simulink model "generalized_plant"  (R2023b)
settings: Solver=VariableStepAuto  StartTime=0.0  StopTime=10.0  RelTol=1e-3
values from neighbouring files (symbols this model uses):
  G_a = 0.095    [Problem_1.m]    (also in Problem_2.m = -0.09; Problem_3.m = 0.014; Problem_4.m = 0.006; Problem_5.m = 0.38)
  G_f = 1 / (K_d*G_s)    (= 1)    [Problem_1.m]    (also in Problem_2.m; Problem_3.m; Problem_4.m; Problem_5.m = 0.125)
  G_s = 1    [Problem_1.m]    (also in Problem_2.m; Problem_3.m; Problem_4.m; Problem_5.m = 2)
libraries: cstblocks x3
settings Model: Creator=vrego  LastModifiedBy=vrego

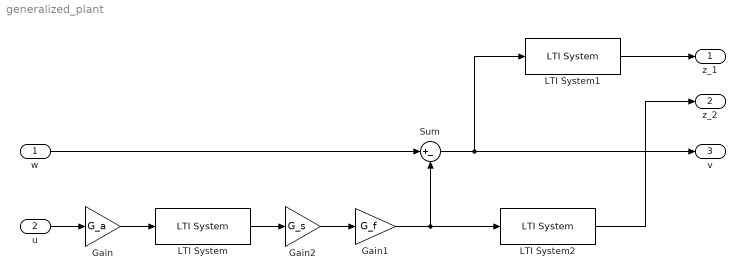
== system generalized_plant ==
  w : Inport
  u : Inport  Port=2
  Gain : Gain  Gain=G_a
  Gain1 : Gain  Gain=G_f
  Gain2 : Gain  Gain=G_s
  LTI System : cstblocks/LTI System  sys=G_pn  IC=[]  PadeOrder=0
  LTI System1 : cstblocks/LTI System  sys=W_1mod  IC=[]  PadeOrder=0
  LTI System2 : cstblocks/LTI System  sys=W_2mod  IC=[]  PadeOrder=0
  Sum : Sum  Inputs=|+-
  z_1 : Outport
  z_2 : Outport  Port=2
  v : Outport  Port=3
  wires:
  Gain/1 -> LTI System/1
  LTI System2/1 -> z_2/1
  Gain1/1 -> Sum/2, LTI System2/1
  Gain2/1 -> Gain1/1
  u/1 -> Gain/1
  Sum/1 -> v/1, LTI System1/1
  w/1 -> Sum/1
  LTI System1/1 -> z_1/1
  LTI System/1 -> Gain2/1
